simulink subsystem "block_sensors"  (R2019b)
settings: Solver=VariableStepAuto  StartTime=0.0  StopTime=10.0  RelTol=1e-3
values from neighbouring files (symbols this model uses):
  A = 0.35    [Sunsensors.m]
  Cs = 1361    [Sunsensors.m]
  low_sat = 0.5    [Sunsensors.m]
  up_sat = 1e4    (= 10000)    [Sunsensors.m]
  var = 1e-4    (= 0.0001)    [Sunsensors.m]
libraries: blocklib x2
settings Model: Creator=imanol  LastModifiedBy=imanol

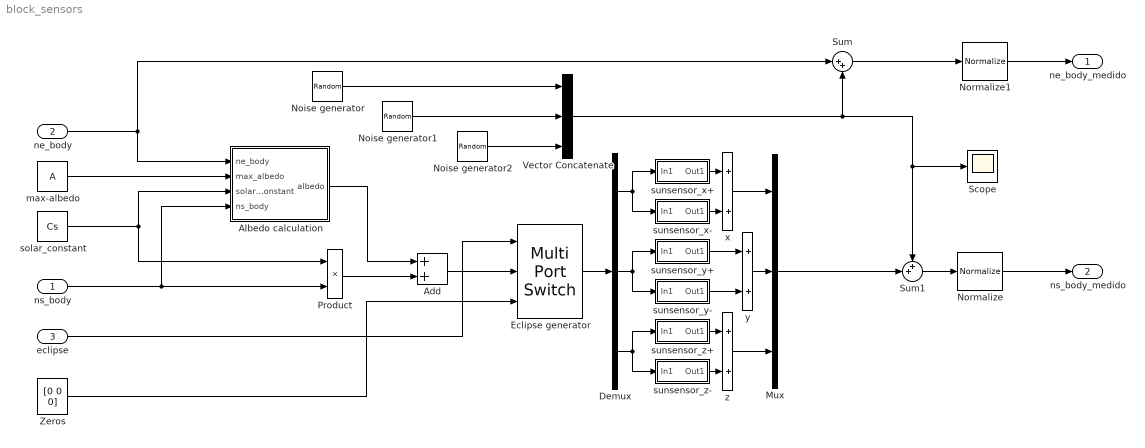
== system block_sensors ==
  ns_body : Inport  PortDimensions=3
  ne_body : Inport  Port=2  PortDimensions=3
  eclipse : Inport  Port=3
  Add : Sum
  Albedo calculation : Subsystem
  Demux : Demux  Outputs=3
  Eclipse generator : MultiPortSwitch  DataPortOrder=Zero-based contiguous  Inputs=2  zeroidx=on
  Mux : Mux  Inputs=3
  Noise generator : RandomNumber  Variance=var  SampleTime=0.1
  Noise generator1 : RandomNumber  Variance=var  Seed=2  SampleTime=0.1
  Noise generator2 : RandomNumber  Variance=var  Seed=3  SampleTime=0.1
  Normalize : blocklib/Normalize  SystemSampleTime=-1  Latency=0  AutoFrameSizeCalculation=off
      settings: SourceProductName=Custom Library
  Normalize1 : blocklib/Normalize  SystemSampleTime=-1  Latency=0  AutoFrameSizeCalculation=off
      settings: SourceProductName=Custom Library
  Product : Product
  Scope : Scope
  Sum : Sum  Inputs=|++
  Sum1 : Sum  Inputs=++|
  Vector Concatenate : Concatenate  NumInputs=3
  Zeros : Constant  Value=[0 0 0]
  max-albedo : Constant  Value=A
  solar_constant : Constant  Value=Cs
  sunsensor_x+ : Subsystem
  sunsensor_x- : Subsystem
  sunsensor_y+ : Subsystem
  sunsensor_y- : Subsystem
  sunsensor_z+ : Subsystem
  sunsensor_z- : Subsystem
  x : Sum
  y : Sum
  z : Sum
  ne_body_medido : Outport  VectorParamsAs1DForOutWhenUnconnected=off
  ns_body_medido : Outport  Port=2  PortDimensions=3  VectorParamsAs1DForOutWhenUnconnected=off
  wires:
  Sum/1 -> Normalize1/1
  sunsensor_z+/1(Out1) -> z/1
  max-albedo/1 -> Albedo calculation/2("max_albedo ")
  ne_body/1 -> Sum/1, Albedo calculation/1(ne_body)
  z/1 -> Mux/3
  Albedo calculation/1(albedo) -> Add/1
  y/1 -> Mux/2
  Mux/1 -> Sum1/2
  sunsensor_z-/1(Out1) -> z/2
  Eclipse generator/1 -> Demux/1
  Demux/3 -> sunsensor_z+/1(In1), sunsensor_z-/1(In1)
  Sum1/1 -> Normalize/1
  Normalize1/1 -> ne_body_medido/1
  sunsensor_y+/1(Out1) -> y/1
  Product/1 -> Add/2
  Demux/2 -> sunsensor_y-/1(In1), sunsensor_y+/1(In1)
  Normalize/1 -> ns_body_medido/1
  sunsensor_x+/1(Out1) -> x/1
  x/1 -> Mux/1
  sunsensor_y-/1(Out1) -> y/2
  sunsensor_x-/1(Out1) -> x/2
  ns_body/1 -> Product/2, Albedo calculation/4(ns_body)
  eclipse/1 -> Eclipse generator/1
  Zeros/1 -> Eclipse generator/3
  solar_constant/1 -> Product/1, Albedo calculation/3(solar_constant)
  Add/1 -> Eclipse generator/2
  Demux/1 -> sunsensor_x+/1(In1), sunsensor_x-/1(In1)
  Noise generator2/1 -> Vector Concatenate/3
  Noise generator1/1 -> Vector Concatenate/2
  Noise generator/1 -> Vector Concatenate/1
  Vector Concatenate/1 -> Sum1/1, Scope/1, Sum/2

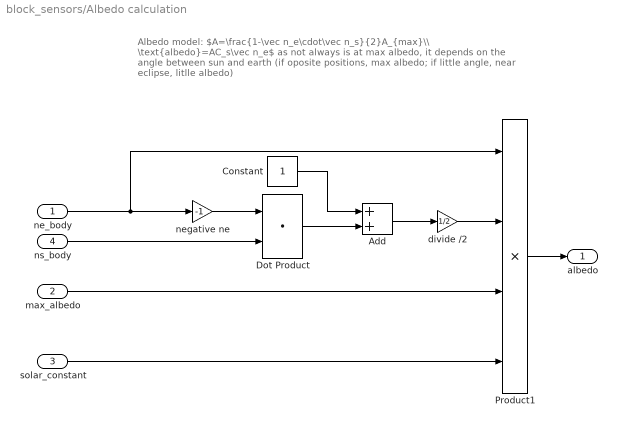
== system block_sensors/Albedo calculation ==
  note: Albedo model:
      | $A=\frac{1-\vec n_e\cdot\vec n_s}{2}A_{max}\\ \text{albedo}=AC_s\vec n_e$
      | as not always is at max albedo, it depends on the angle between sun and earth
      | (if oposite positions, max albedo; if little angle, near eclipse, litlle albedo)
  ne_body : Inport
  "max_albedo " : Inport  Port=2
  solar_constant : Inport  Port=3
  ns_body : Inport  Port=4
  Add : Sum
  Constant : Constant
  Dot Product : DotProduct  InputSameDT=on  OutDataTypeStr=Inherit: Inherit via internal rule
  Product1 : Product  Inputs=4
  divide /2 : Gain  Gain=1/2
  negative ne : Gain  Gain=-1
  albedo : Outport  VectorParamsAs1DForOutWhenUnconnected=off
  wires:
  Product1/1 -> albedo/1
  solar_constant/1 -> Product1/4
  negative ne/1 -> Dot Product/1
  ns_body/1 -> Dot Product/2
  ne_body/1 -> Product1/1, negative ne/1
  "max_albedo "/1 -> Product1/3
  Dot Product/1 -> Add/2
  Add/1 -> divide /2/1
  Constant/1 -> Add/1
  divide /2/1 -> Product1/2

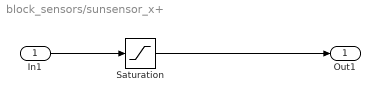
== system block_sensors/sunsensor_x+ ==
  In1 : Inport
  Saturation : Saturate  UpperLimit=up_sat  LowerLimit=low_sat
  Out1 : Outport  VectorParamsAs1DForOutWhenUnconnected=off
  wires:
  In1/1 -> Saturation/1
  Saturation/1 -> Out1/1

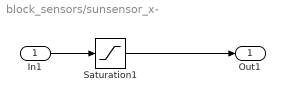
== system block_sensors/sunsensor_x- ==
  In1 : Inport
  Saturation1 : Saturate  UpperLimit=-low_sat  LowerLimit=-up_sat
  Out1 : Outport  VectorParamsAs1DForOutWhenUnconnected=off
  wires:
  In1/1 -> Saturation1/1
  Saturation1/1 -> Out1/1

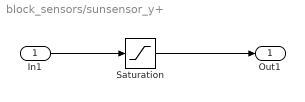
== system block_sensors/sunsensor_y+ ==
  In1 : Inport
  Saturation : Saturate  UpperLimit=up_sat  LowerLimit=low_sat
  Out1 : Outport  VectorParamsAs1DForOutWhenUnconnected=off
  wires:
  In1/1 -> Saturation/1
  Saturation/1 -> Out1/1

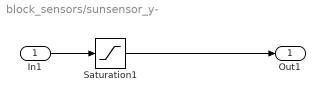
== system block_sensors/sunsensor_y- ==
  In1 : Inport
  Saturation1 : Saturate  UpperLimit=-low_sat  LowerLimit=-up_sat
  Out1 : Outport  VectorParamsAs1DForOutWhenUnconnected=off
  wires:
  In1/1 -> Saturation1/1
  Saturation1/1 -> Out1/1

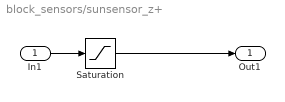
== system block_sensors/sunsensor_z+ ==
  In1 : Inport
  Saturation : Saturate  UpperLimit=up_sat  LowerLimit=low_sat
  Out1 : Outport  VectorParamsAs1DForOutWhenUnconnected=off
  wires:
  In1/1 -> Saturation/1
  Saturation/1 -> Out1/1

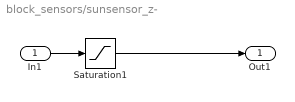
== system block_sensors/sunsensor_z- ==
  In1 : Inport
  Saturation1 : Saturate  UpperLimit=-low_sat  LowerLimit=-up_sat
  Out1 : Outport  VectorParamsAs1DForOutWhenUnconnected=off
  wires:
  In1/1 -> Saturation1/1
  Saturation1/1 -> Out1/1
